simulink model "proof_simulink_trajectory"  (R2019b)
settings: Solver=ode45  StartTime=0.0  StopTime=5  RelTol=1e-3  EnableMultiTasking=on
libraries: simulink x1
settings Model: Creator=CR7  LastModifiedBy=user
settings DataIOCC: LimitDataPoints=on  SaveFormat=Array  ReturnWorkspaceOutputs=off
settings OptimizationCC: LifeSpan=inf
settings DebuggingCC: SFUnexpectedBacktrackingDiag=warning  SFNoUnconditionalDefaultTransitionDiag=warning  SFExecutionAtInitializationDiag=none  ArithmeticOperatorsInVariantConditions=warning
settings HardwareCC: ProdBitPerPointer=32  ProdBitPerSizeT=32  ProdBitPerPtrDiffT=32  ProdLargestAtomicFloat=None  ProdIntDivRoundTo=Undefined  ProdEndianess=Unspecified  ProdWordSize=32  ProdHWDeviceType=32-bit Generic
settings ModelReferenceCC: PropagateSignalLabelsOutOfModel=off
settings SFSimCC: SimUseLocalCustomCode=off  CustomCodeUndefinedFunction=UseInterfaceOnly
settings RTWCC: RTWUseLocalCustomCode=off
settings CodeAppCC: StateflowObjectComments=on
settings GRTTargetCC: TargetLangStandard=C89/C90 (ANSI)  GeneratePreprocessorConditionals=Disable all
settings ConfigComp: CovMetricSettings=dw  CovHtmlReporting=on  CovSaveCumulativeToWorkspaceVar=on  CovSaveSingleToWorkspaceVar=on  CovExternalEMLEnable=off

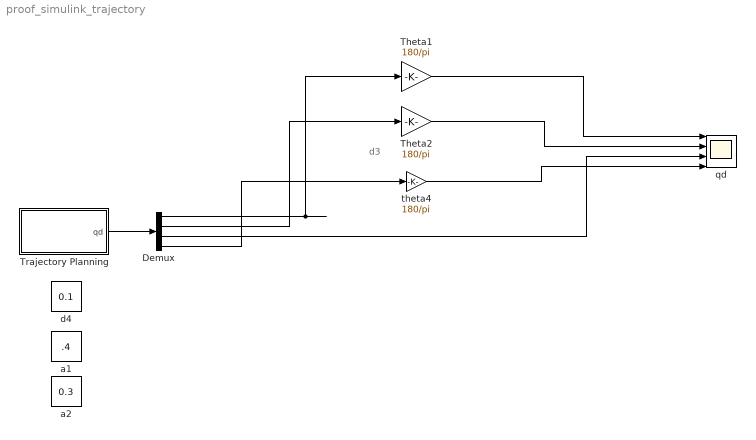
== system proof_simulink_trajectory ==
  note: d3
  Demux : Demux
  Theta1 : Gain  Gain=180/pi
  Theta2 : Gain  Gain=180/pi
  Trajectory Planning : Subsystem
  a1 : Constant  Value=.4
  a2 : Constant  Value=0.3
  d4 : Constant  Value=0.1
  qd : Scope  NumInputPorts=4
  theta4 : Gain  Gain=180/pi
  wires:
  Theta1/1 -> qd/1
  Theta2/1 -> qd/2
  Trajectory Planning/1(qd) -> Demux/1
  theta4/1 -> qd/4
  Demux/1 -> Theta1/1
  Demux/2 -> Theta2/1
  Demux/3 -> qd/3
  Demux/4 -> theta4/1

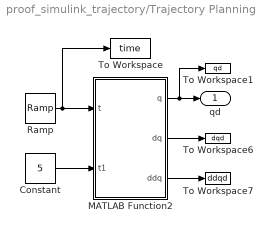
== system proof_simulink_trajectory/Trajectory Planning ==
  Constant : Constant  Value=5
  MATLAB Function2 : MATLAB Function  TreatAsAtomicUnit=on
  Ramp : simulink/Sources/Ramp  slope=1  start=0  InitialOutput=0
  To Workspace : ToWorkspace  VariableName=time  SampleTime=-1
  To Workspace1 : ToWorkspace  VariableName=qd  SampleTime=-1
  To Workspace6 : ToWorkspace  VariableName=dqd  SampleTime=-1
  To Workspace7 : ToWorkspace  VariableName=ddqd  SampleTime=-1
  qd : Outport
  wires:
  MATLAB Function2/1(q) -> To Workspace1/1, qd/1
  Ramp/1 -> To Workspace/1, MATLAB Function2/1(t)
  Constant/1 -> MATLAB Function2/2(t1)
  MATLAB Function2/2(dq) -> To Workspace6/1
  MATLAB Function2/3(ddq) -> To Workspace7/1

== matlab function proof_simulink_trajectory/Trajectory Planning/MATLAB Function2 ==
  data: t input; q output; dq output; ddq output; t1 input
function [q,dq,ddq] = fcn(t,t1)
%#codegen
t1 = t/t1;
q0 = [(0)*pi/180;(0)*pi/180;(0);(0)*pi/180];
qf = [(90)*pi/180;(30)*pi/180;(0.1);(180)*pi/180];

q = q0 + 3*(qf-q0)*t1^2 - 2*(qf-q0)*t1^3;
dq = 6*(qf-q0)*t1 - 6*(qf-q0)*t1^2;
ddq = 6*(qf-q0) - 12*(qf-q0)*t1;
% q
% t1

% a   = [ 32.5*pi/180; 45*pi/180];
% w   = [ pi/3; pi/2];
% q   = a.*(  sin(w.*t) );
% dq  = a.*(  w.*cos(w.*t) );
% ddq = a.*( -w.*w.*sin(w.*t) );
% 
% 
% q   = q + [(45)*pi/180;pi/2];

% % if t>5
%     q = [(45)*pi/180;pi/2];
%     dq  = [0,0]';
%     ddq = [0,0]';
% % end
